simulink model "BirdHeadModelControlled_MovementControl"  (R2023a)
settings: Solver=FixedStepAuto  StartTime=0.0  StopTime=tsim  FixedStep=dt  RelTol=1e-3
values from neighbouring files (symbols this model uses):
  amplitude_gamma = deg2rad(-10)    [LaunchBirdHeadModelControlled_MovementControl.m]    (also in PlotMovementControl.m)
  amplitude_theta = deg2rad(10)    [LaunchBirdHeadModelControlled_MovementControl.m]    (also in PlotMovementControl.m)
  dt = 0.002    [LaunchBirdHeadModel2.m]    (also in LaunchBirdHeadModelControlled.m; LaunchBirdHeadModelControlled_MovementControl.m; PlotMovementControl.m; PlotPositionControl.m)
  f = frequencies(k)    [LaunchBirdHeadModelControlled_MovementControl.m]    (also in PlotMovementControl.m = 0.25)
  g = 9.81    [LaunchBirdHeadModel2.m]    (also in LaunchBirdHeadModelControlled.m; LaunchBirdHeadModelControlled_MovementControl.m; PlotMovementControl.m; PlotPositionControl.m)
  gamma_init = init_cond(j,2)    [LaunchBirdHeadModelControlled_MovementControl.m]    (also in PlotMovementControl.m = deg2rad(0))
  I_by = 0.00001    (= 1e-05)    [LaunchBirdHeadModel2.m]    (also in LaunchBirdHeadModelControlled.m; LaunchBirdHeadModelControlled_MovementControl.m; PlotMovementControl.m; PlotPositionControl.m)
  I_hy = 0.00001    (= 1e-05)    [LaunchBirdHeadModel2.m]    (also in LaunchBirdHeadModelControlled.m; LaunchBirdHeadModelControlled_MovementControl.m; PlotMovementControl.m; PlotPositionControl.m)
  Kp = [20  0; 0  20]    [CondIni-1010Kp201Kv101.mat]    (also in Kp101Kv51.mat = [20  0; 0  1]; Kp11Kv051.mat = [1  0; 0  1]; Kp11Kv11.mat = [1  0; 0  1]; Kp11Kv21.mat = [1  0; 0  1])
  Kv = [10  0; 0  10]    [CondIni-1010Kp201Kv101.mat]    (also in Kp101Kv51.mat = [5  0; 0  1]; Kp11Kv051.mat = [0.5  0; 0  1]; Kp11Kv11.mat = [1  0; 0  1]; Kp11Kv21.mat = [2  0; 0  1])
  l_b = 0.05    [LaunchBirdHeadModel2.m]    (also in LaunchBirdHeadModelControlled.m; LaunchBirdHeadModelControlled_MovementControl.m; PlotMovementControl.m; PlotPositionControl.m)
  l_ec = 0.020    (= 0.02)    [LaunchBirdHeadModelControlled_MovementControl.m]    (also in PlotMovementControl.m; PlotPositionControlWS.mat)
  l_h = 0.04    [LaunchBirdHeadModel2.m]    (also in LaunchBirdHeadModelControlled.m; LaunchBirdHeadModelControlled_MovementControl.m; PlotMovementControl.m; PlotPositionControl.m)
  m_h = 0.005    [LaunchBirdHeadModel2.m]    (also in LaunchBirdHeadModelControlled.m; LaunchBirdHeadModelControlled_MovementControl.m; PlotMovementControl.m; PlotPositionControl.m)
  theta_init = init_cond(j,1)    [LaunchBirdHeadModelControlled_MovementControl.m]    (also in PlotMovementControl.m = deg2rad(0))
libraries: simulink_extras x4
settings Model: Creator=coquet  LastModifiedBy=coquet

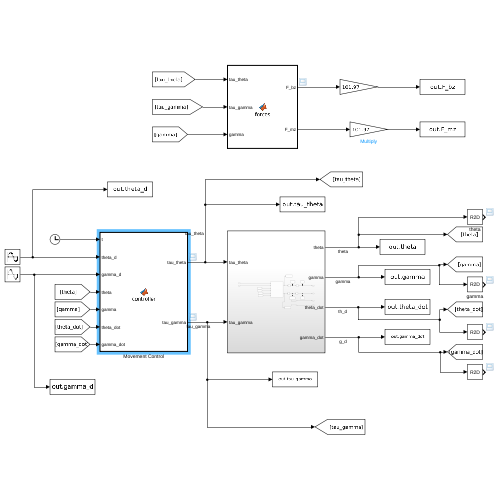
[thumbnail: Simulink's stored preview of the top-level diagram]
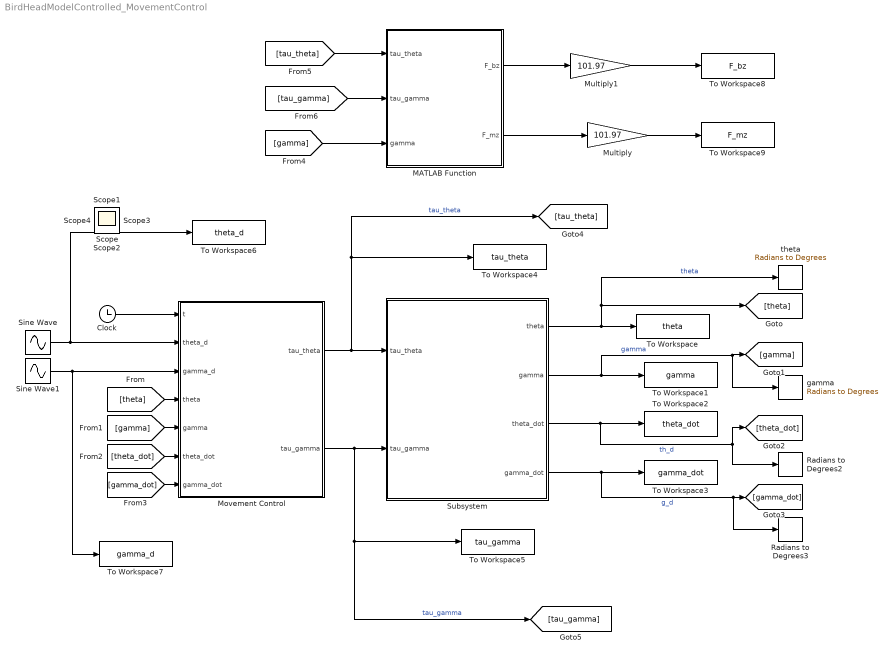
== system BirdHeadModelControlled_MovementControl ==
  Clock : Clock
  MATLAB Function : MATLAB Function  TreatAsAtomicUnit=on
  Movement Control : MATLAB Function  TreatAsAtomicUnit=on
  Multiply : Gain  Gain=101.97
  Multiply1 : Gain  Gain=101.97
  Radians to Degrees2 : simulink_extras/Transformations/Radians to Degrees
  Radians to Degrees3 : simulink_extras/Transformations/Radians to Degrees
  Sine Wave : Sin  Amplitude=deg2rad(10)  Frequency=2*pi*f  SampleTime=dt
  Sine Wave1 : Sin  Amplitude=-deg2rad(10)  SampleTime=dt
  Subsystem : Subsystem
  To Workspace : ToWorkspace  VariableName=theta  SaveFormat=Timeseries  SampleTime=dt
  To Workspace1 : ToWorkspace  VariableName=gamma  SaveFormat=Timeseries  SampleTime=dt
  To Workspace2 : ToWorkspace  VariableName=theta_dot  SaveFormat=Timeseries  SampleTime=dt
  To Workspace3 : ToWorkspace  VariableName=gamma_dot  SaveFormat=Timeseries  SampleTime=dt
  To Workspace4 : ToWorkspace  VariableName=tau_theta  SaveFormat=Timeseries  SampleTime=dt
  To Workspace5 : ToWorkspace  VariableName=tau_gamma  SaveFormat=Timeseries  SampleTime=dt
  To Workspace6 : ToWorkspace  VariableName=theta_d  SaveFormat=Timeseries  SampleTime=dt
  To Workspace7 : ToWorkspace  VariableName=gamma_d  SaveFormat=Timeseries  SampleTime=dt
  To Workspace8 : ToWorkspace  VariableName=F_bz  SaveFormat=Timeseries  SampleTime=dt
  To Workspace9 : ToWorkspace  VariableName=F_mz  SaveFormat=Timeseries  SampleTime=dt
  gamma : simulink_extras/Transformations/Radians to Degrees
  theta : simulink_extras/Transformations/Radians to Degrees
  Scope{,1..4} (5 alike) : Scope
  wires:
  Subsystem/4(gamma_dot) -> To Workspace3/1, Radians to Degrees3/1, [gamma_dot]  "g_d"
  Subsystem/1(theta) -> theta/1, [theta], To Workspace/1  "theta"
  Subsystem/3(theta_dot) -> Radians to Degrees2/1, [theta_dot], To Workspace2/1  "th_d"
  Subsystem/2(gamma) -> gamma/1, [gamma], To Workspace1/1  "gamma"
  [theta] -> Movement Control/4(theta)
  [gamma] -> Movement Control/5(gamma)
  [theta_dot] -> Movement Control/6(theta_dot)
  [gamma_dot] -> Movement Control/7(gamma_dot)
  Movement Control/1(tau_theta) -> [tau_theta], To Workspace4/1, Subsystem/1(tau_theta)  "tau_theta"
  Movement Control/2(tau_gamma) -> [tau_gamma], To Workspace5/1, Subsystem/2(tau_gamma)  "tau_gamma"
  Sine Wave/1 -> To Workspace6/1, Movement Control/2(theta_d)
  Sine Wave1/1 -> To Workspace7/1, Movement Control/3(gamma_d)
  Clock/1 -> Movement Control/1(t)
  [gamma] -> MATLAB Function/3(gamma)
  [tau_theta] -> MATLAB Function/1(tau_theta)
  [tau_gamma] -> MATLAB Function/2(tau_gamma)
  MATLAB Function/2(F_mz) -> Multiply/1
  Multiply/1 -> To Workspace9/1
  MATLAB Function/1(F_bz) -> Multiply1/1
  Multiply1/1 -> To Workspace8/1

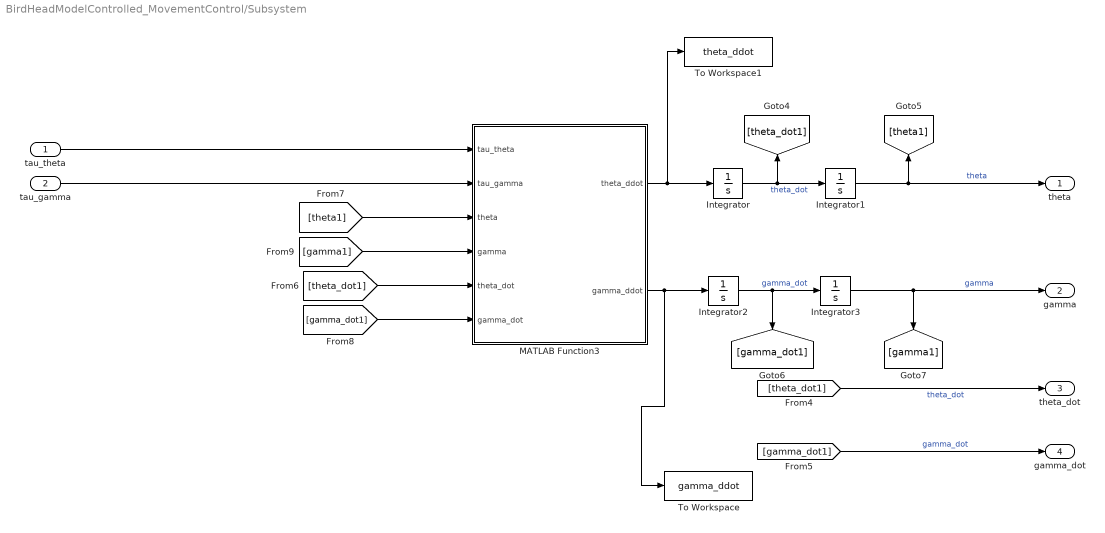
== system BirdHeadModelControlled_MovementControl/Subsystem ==
  tau_theta : Inport
  tau_gamma : Inport  Port=2
  Integrator : Integrator  ContinuousStateAttributes='theta_dot'
  Integrator1 : Integrator  InitialCondition=theta_init  UpperSaturationLimit=2*pi/9  LowerSaturationLimit=-pi/3  WrapState=on  ContinuousStateAttributes='theta'
  Integrator2 : Integrator  ContinuousStateAttributes='gamma_dot'
  Integrator3 : Integrator  InitialCondition=gamma_init  UpperSaturationLimit=2*pi/9  LowerSaturationLimit=-pi/3  WrapState=on  ContinuousStateAttributes='gamma'
  MATLAB Function3 : MATLAB Function  TreatAsAtomicUnit=on
  To Workspace : ToWorkspace  VariableName=gamma_ddot  SaveFormat=Timeseries  SampleTime=-1
  To Workspace1 : ToWorkspace  VariableName=theta_ddot  SaveFormat=Timeseries  SampleTime=-1
  theta : Outport
  gamma : Outport  Port=2
  theta_dot : Outport  Port=3
  gamma_dot : Outport  Port=4
  wires:
  [gamma1] -> MATLAB Function3/4(gamma)
  Integrator1/1 -> theta/1, [theta1]  "theta"
  [theta1] -> MATLAB Function3/3(theta)
  tau_theta/1 -> MATLAB Function3/1(tau_theta)
  [theta_dot1] -> MATLAB Function3/5(theta_dot)
  MATLAB Function3/1(theta_ddot) -> To Workspace1/1, Integrator/1
  [gamma_dot1] -> MATLAB Function3/6(gamma_dot)
  [theta_dot1] -> theta_dot/1  "theta_dot"
  MATLAB Function3/2(gamma_ddot) -> To Workspace/1, Integrator2/1
  Integrator3/1 -> gamma/1, [gamma1]  "gamma"
  tau_gamma/1 -> MATLAB Function3/2(tau_gamma)
  Integrator2/1 -> [gamma_dot1], Integrator3/1  "gamma_dot"
  [gamma_dot1] -> gamma_dot/1  "gamma_dot"
  Integrator/1 -> Integrator1/1, [theta_dot1]  "theta_dot"

== matlab function BirdHeadModelControlled_MovementControl/MATLAB Function ==
  data: tau_theta input; F_bz output; tau_gamma input; gamma input; l_ec parameter; l_h parameter; F_mz output; l_b parameter
function [F_bz,F_mz] = forces(tau_theta, tau_gamma, gamma, l_ec, l_h, l_b)

tau = [tau_theta; tau_gamma];

% tau = [l_ec, l_h*cos(gamma)+l_ec; l_ej*cos(gamma), l_m] * F;

F = [l_ec, -l_b*cos(gamma)-l_h; 0, -l_h] \ tau;

F_bz = F(1);
F_mz = F(2)/cos(deg2rad(10));

== matlab function BirdHeadModelControlled_MovementControl/Movement Control ==
  data: t input; tau_theta output; theta_d input; gamma_d input; theta input; gamma input; theta_dot input; gamma_dot input; Kv parameter; Kp parameter; I_hy parameter; I_by parameter; l_h parameter; l_b parameter; m_h parameter; g parameter; tau_gamma output; f parameter; amplitude_theta parameter; amplitude_gamma parameter
function [tau_theta, tau_gamma] = controller(t, theta_d, gamma_d, theta, gamma, theta_dot, gamma_dot, Kv, Kp, I_hy, I_by, l_h, l_b, m_h, g, f, amplitude_theta, amplitude_gamma)

theta_d = amplitude_theta*sin(2*pi*f*t);
theta_dot_d = amplitude_theta*(2*pi*f)*cos(2*pi*f*t);
theta_ddot_d = -amplitude_theta*(2*pi*f)^2*sin(2*pi*f*t);

gamma_d = amplitude_gamma*sin(2*pi*f*t);
gamma_dot_d = amplitude_gamma*(2*pi*f)*cos(2*pi*f*t);
gamma_ddot_d = -amplitude_gamma*(2*pi*f)^2*sin(2*pi*f*t);



m11 = I_hy+I_by+m_h*(l_b^2+l_h^2)+2*l_b*l_h*m_h*cos(gamma);
m12 = I_hy+m_h*l_h^2+l_b*l_h*m_h*cos(gamma);
m22 = I_hy + l_h^2*m_h;

M=[m11 m12;
   m12 m22];


c11 = -l_b*l_h*m_h*sin(gamma)*gamma_dot;
c12 = -(gamma_dot+theta_dot)*l_b*l_h*m_h*sin(gamma);
c21 = l_b*l_h*m_h*sin(gamma)*theta_dot;
c22 = 0;

C=[c11 c12; 
   c21 c22];

g1 = -g*m_h*cos(theta)*(l_b+l_h*cos(gamma))+g*l_h*m_h*sin(gamma)*sin(theta);
g2 = -l_h*m_h*cos(gamma+theta)*g;

G=[g1;g2];

%% Desired model
m11_d = I_hy+I_by+m_h*(l_b^2+l_h^2)+2*l_b*l_h*m_h*cos(gamma_d);
m12_d = I_hy+m_h*l_h^2+l_b*l_h*m_h*cos(gamma_d);
m22_d = I_hy + l_h^2*m_h;

M_d=[m11_d m12_d;
   m12_d m22_d];


c11_d = -l_b*l_h*m_h*sin(gamma_d)*gamma_dot_d;
c12_d = -(gamma_dot_d+theta_dot_d)*l_b*l_h*m_h*sin(gamma_d);
c21_d = l_b*l_h*m_h*sin(gamma_d)*theta_dot_d;
c22_d = 0;

C_d=[c11_d c12_d; 
   c21_d c22_d];

g1_d = -g*m_h*cos(theta_d)*(l_b+l_h*cos(gamma_d))+g*l_h*m_h*sin(gamma_d)*sin(theta_d);
g2_d = -l_h*m_h*cos(gamma_d+theta_d)*g;

G_d=[g1_d;g2_d];

%% Controlled Torque

tau = M*(Kp*[theta_d-theta;gamma_d-gamma] + Kv*[theta_dot_d - theta_dot;gamma_dot_d - gamma_dot]) + M_d*[theta_ddot_d; gamma_ddot_d] + C_d*[theta_dot_d; gamma_dot_d] + G_d;

tau_theta = tau(1);
tau_gamma = tau(2);

== matlab function BirdHeadModelControlled_MovementControl/Subsystem/MATLAB Function3 ==
  data: tau_theta input; tau_gamma input; theta_ddot output; theta input; gamma input; theta_dot input; gamma_dot input; gamma_ddot output; I_hy parameter; m_h parameter; l_b parameter; l_h parameter; I_by parameter; g parameter
function [theta_ddot, gamma_ddot] = fcn(tau_theta, tau_gamma,theta,gamma,theta_dot,gamma_dot, I_hy, m_h, l_b, l_h, I_by,g)

tau = [tau_theta;tau_gamma];

m11 = I_hy+I_by+m_h*(l_b^2+l_h^2)+2*l_b*l_h*m_h*cos(gamma);
m12 = I_hy+m_h*l_h^2+l_b*l_h*m_h*cos(gamma);
m22 = I_hy + l_h^2*m_h;

M=[m11 m12;
   m12 m22];


c11 = -l_b*l_h*m_h*sin(gamma)*gamma_dot;
c12 = -(gamma_dot+theta_dot)*l_b*l_h*m_h*sin(gamma);
c21 = l_b*l_h*m_h*sin(gamma)*theta_dot;
c22 = 0;

C=[c11 c12; 
   c21 c22];

g1 = -g*m_h*cos(theta)*(l_b+l_h*cos(gamma))+g*l_h*m_h*sin(gamma)*sin(theta);
g2 = -l_h*m_h*cos(gamma+theta)*g;

G=[g1;g2];

qddot=M\(tau-C*[theta_dot;gamma_dot]-G);

theta_ddot=qddot(1);
gamma_ddot=qddot(2);
